simulink model "WiperSystem"  (R2023a)
settings: Solver=FixedStepDiscrete  StartTime=0.0  StopTime=20  FixedStep=0.001  RelTol=1e-3  EnableMultiTasking=on
undefined symbols (not defined in the file): sigbuilder_block
libraries: arduinolib x2, simulink x1
settings Model: ExtModeTrigDuration=2  Creator=waleed.elshemy  LastModifiedBy=Youssef Ait Mouna
settings SolverCC: AutoInsertRateTranBlk=on
settings OptimizationCC: UseDivisionForNetSlopeComputation=on  GainParamInheritBuiltInType=on  UseFloatMulNetSlope=on  PassReuseOutputArgsAs=Individual arguments  ZeroExternalMemoryAtStartup=off  ZeroInternalMemoryAtStartup=off  NoFixptDivByZeroProtection=on  EfficientFloat2IntCast=on  LifeSpan=1  MaxStackSize=64  OptimizeBlockOrder=speed  DifferentSizesBufferReuse=on  EfficientTunableParamExpr=on
settings DebuggingCC: ParameterTunabilityLossMsg=error  UnconnectedInputMsg=warning  UnconnectedOutputMsg=warning  UnconnectedLineMsg=warning
settings HardwareCC: ProdBitPerInt=16  ProdBitPerPointer=16  ProdBitPerSizeT=16  ProdBitPerPtrDiffT=16  ProdLargestAtomicFloat=None  ProdWordSize=8  ProdHWDeviceType=Atmel->AVR
settings ModelReferenceCC: EnableRefExpFcnMdlSchedulingChecks=on
settings SFSimCC: MATLABDynamicMemAlloc=off
settings RTWCC: Description=Embedded Coder  SystemTargetFile=ert.tlc  HardwareBoard=Arduino Uno  TemplateMakefile=ert_default_tmf  Toolchain=Arduino AVR  BuildConfiguration=Faster Runs  DLArmComputeVersion=19.05
settings CodeAppCC: ForceParamTrailComments=on  IgnoreCustomStorageClasses=off  OperatorAnnotations=on  SimulinkDataObjDesc=on  SFDataObjDesc=on  CustomSymbolStrGlobalVar=rt$N$M  CustomSymbolStrType=$N$M  CustomSymbolStrFcn=$N$M$F  CustomSymbolStrMacro=$N$M  InsertBlockDesc=on
settings ERTTargetCC: IncludeMdlTerminateFcn=off  CombineSignalStateStructs=on  SupportComplex=off  SupportContinuousTime=on  SupportNonInlinedSFcns=on  SupportVariableSizeSignals=on  ExtModeTransport=3  ExtModeStaticAlloc=on  ExtModeAutomaticAllocSize=off  ExtModeStaticAllocSize=250  ExtModeMexFile=ext_xcp  ExtModeIntrfLevel=Level2 - Open  ERTFilePackagingFormat=CompactWithDataFile

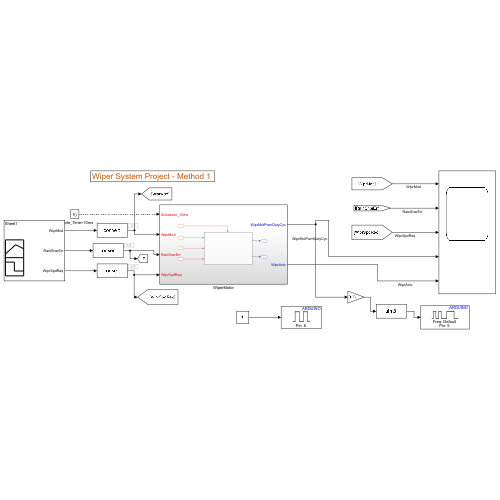
[thumbnail: Simulink's stored preview of the top-level diagram]
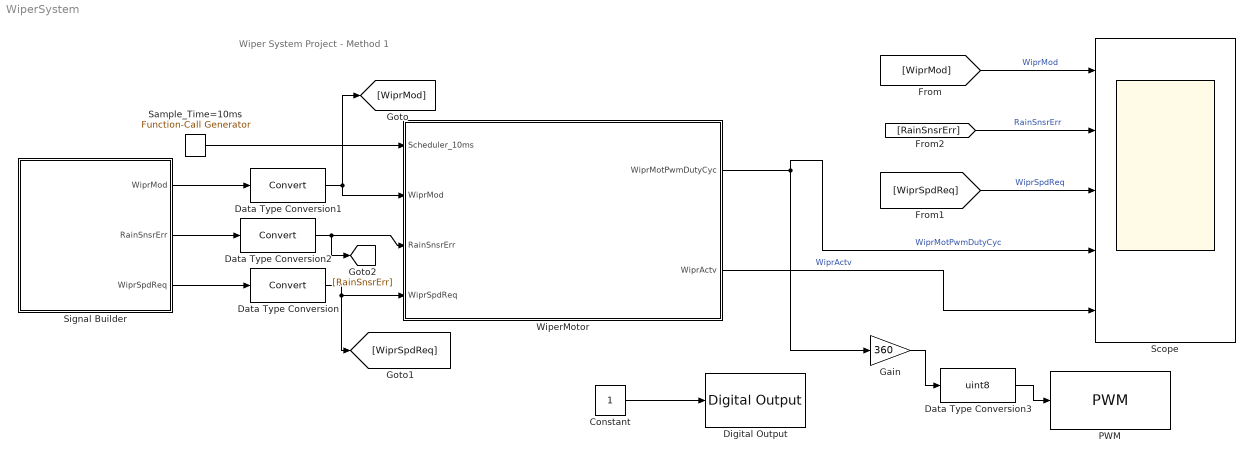
== system WiperSystem ==
  note: Wiper System Project - Method 1
  Constant : Constant
  Data Type Conversion : DataTypeConversion  SaturateOnIntegerOverflow=off  RndMeth=Floor
  Data Type Conversion1 : DataTypeConversion  SaturateOnIntegerOverflow=off  RndMeth=Floor
  Data Type Conversion2 : DataTypeConversion  SaturateOnIntegerOverflow=off  RndMeth=Floor
  Data Type Conversion3 : DataTypeConversion  OutDataTypeStr=uint8  SaturateOnIntegerOverflow=off  RndMeth=Floor
  Digital Output : arduinolib/Digital Output  pinNumber=6  Direction=output  blockPlatform=arduino
  Gain : Gain  Gain=360  OutDataTypeStr=uint8
  PWM : arduinolib/PWM  pinNumber=5  frequencyType=Default  desiredFrequency=490.2  achievableFrequency=490.2
  Sample_Time=10ms : simulink/Ports & Subsystems/Function-Call Generator  sample_time=0.01  numberOfIterations=1  DisallowWideOutput=off
  Scope : Scope  NumInputPorts=5
  Signal Builder : Subsystem  Tag=STV Subsys  LoadFcn=sigbuilder_block('load');  StartFcn=sigbuilder_block('start');  StopFcn=sigbuilder_block('stop');  ClipboardFcn=sigbuilder_block('clipboard');  mask(Sigbuilder block){tuvar=[0:10]}
      mask help: Simulink:masks:SigbuilderBlock_MD
      mask init:
      | if ~strcmp(get_param(bdroot(gcbh),'SimulationStatus'),'stopped') tuvar = sigbuilder_block('maskInit'); end
      settings: CopyFcn=sigbuilder_block('copy');  DeleteFcn=sigbuilder_block('delete');  ModelCloseFcn=sigbuilder_block('modelClose');  PreSaveFcn=sigbuilder_block('preSave');  PauseFcn=sigbuilder_block('pause');  ContinueFcn=sigbuilder_block('continue');  NameChangeFcn=sigbuilder_block('namechange');  OpenFcn=sigbuilder_block('open',[547.2 117.6 550.8 362.4 ]);  CloseFcn=sigbuilder_block('close');
      mask Display: plot(0, 0, 100, 100,[2, 2, 32, 32, 2], [68, 8, 8, 68, 68],[32, 2], [38, 38], [32, 19, 2],[53, 60, 44], [32, 17, 17, 2],[16, 16, 31, 31]);txt = getActiveGroup(gcbh);text(2, 100, txt,'verticalAlignment', 'top');
  WiperMotor : Subsystem
  wires:
  Sample_Time=10ms/1 -> WiperMotor/1(Scheduler_10ms)
  WiperMotor/1(WiprMotPwmDutyCyc) -> Scope/4, Gain/1  "WiprMotPwmDutyCyc"
  WiperMotor/2(WiprActv) -> Scope/5  "WiprActv"
  Signal Builder/1(WiprMod) -> Data Type Conversion1/1
  Signal Builder/3(WiprSpdReq) -> Data Type Conversion/1
  Data Type Conversion/1 -> [WiprSpdReq], WiperMotor/4(WiprSpdReq)
  Data Type Conversion1/1 -> [WiprMod], WiperMotor/2(WiprMod)
  [WiprMod] -> Scope/1  "WiprMod"
  Data Type Conversion2/1 -> [RainSnsrErr], WiperMotor/3(RainSnsrErr)
  Signal Builder/2(RainSnsrErr) -> Data Type Conversion2/1
  [WiprSpdReq] -> Scope/3  "WiprSpdReq"
  [RainSnsrErr] -> Scope/2  "RainSnsrErr"
  Constant/1 -> Digital Output/1
  Gain/1 -> Data Type Conversion3/1
  Data Type Conversion3/1 -> PWM/1

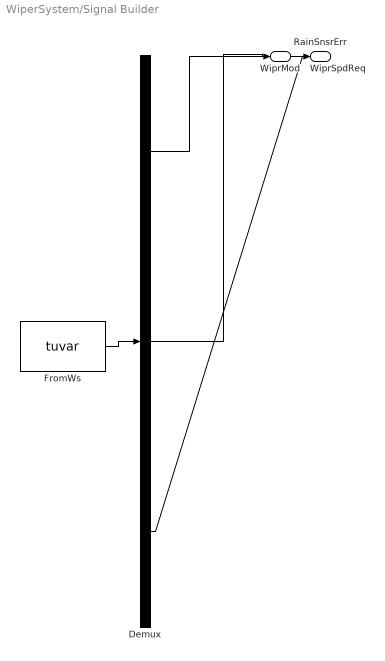
== system WiperSystem/Signal Builder ==
  Demux : Demux  Tag=STV Demux  Outputs=3
      settings: DisplayOption=none
  FromWs : FromWorkspace  Tag=STV FromWs  VariableName=tuvar  SampleTime=1  OutputAfterFinalValue=Holding final value
      SigBuilderData=|
      | common.afterFinalStr = 'Hold final value'
      | common.sampleTime = '1'
      | dataSet.timeRange = [0 16]
      | dataSet.name = 'Sheet1'
      | sbobj.Groups.Name = 'Sheet1'
      | sbobj.Groups.Signals(1).Name = 'WiprMod'
      | sbobj.Groups.Signals(1).XData = [0 1 2 3 4 5 6 7 8 9 10 11 12 13 14 15 16]
      | sbobj.Groups.Signals(1).YData = [0 0 2 2 3 3 1 1 1 1 1 1 1 1 1 1 1]
      | sbobj.Groups.Signals(2).Name = 'RainSnsrErr'
      | sbobj.Groups.Signals(2).XData = [0 1 2 3 4 5 6 7 8 9 10 11 12 13 14 15 16]
      | sbobj.Groups.Signals(2).YData = [0 0 0 0 0 0 0 0 0 0 0 0 0 0 0 1 0]
      | sbobj.Groups.Signals(3).Name = 'WiprSpdReq'
      | sbobj.Groups.Signals(3).XData = [0 1 2 3 4 5 6 7 8 9 10 11 12 13 14 15 16]
      | sbobj.Groups.Signals(3).YData = [0 0 0 0 0 0 0 0 1 2 3 4 5 6 7 7 7]
      | sbobj.Groups.TimeRange = [0 16]
  WiprMod : Outport  Tag=STV Outport
  RainSnsrErr : Outport  Tag=STV Outport  Port=2
  WiprSpdReq : Outport  Tag=STV Outport  Port=3
  wires:
  Demux/1 -> WiprMod/1
  FromWs/1 -> Demux/1
  Demux/2 -> RainSnsrErr/1
  Demux/3 -> WiprSpdReq/1

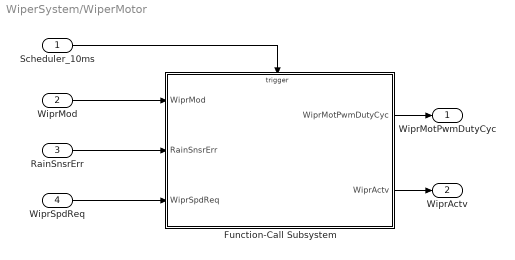
== system WiperSystem/WiperMotor ==
  Scheduler_10ms : Inport
  WiprMod : Inport  Port=2  OutMin=0  OutMax=3  OutDataTypeStr=uint8
  RainSnsrErr : Inport  Port=3  OutMin=0  OutMax=1  OutDataTypeStr=boolean
  WiprSpdReq : Inport  Port=4  OutMin=0  OutMax=7  OutDataTypeStr=uint8
  Function-Call Subsystem : Subsystem  TreatAsAtomicUnit=on
  WiprMotPwmDutyCyc : Outport  OutMin=0  OutMax=1  OutDataTypeStr=single  LockScale=on
  WiprActv : Outport  Port=2  OutDataTypeStr=boolean
  wires:
  WiprMod/1 -> Function-Call Subsystem/1(WiprMod)
  WiprSpdReq/1 -> Function-Call Subsystem/3(WiprSpdReq)
  Function-Call Subsystem/2(WiprActv) -> WiprActv/1
  Scheduler_10ms/1 -> Function-Call Subsystem/Trigger
  RainSnsrErr/1 -> Function-Call Subsystem/2(RainSnsrErr)
  Function-Call Subsystem/1(WiprMotPwmDutyCyc) -> WiprMotPwmDutyCyc/1

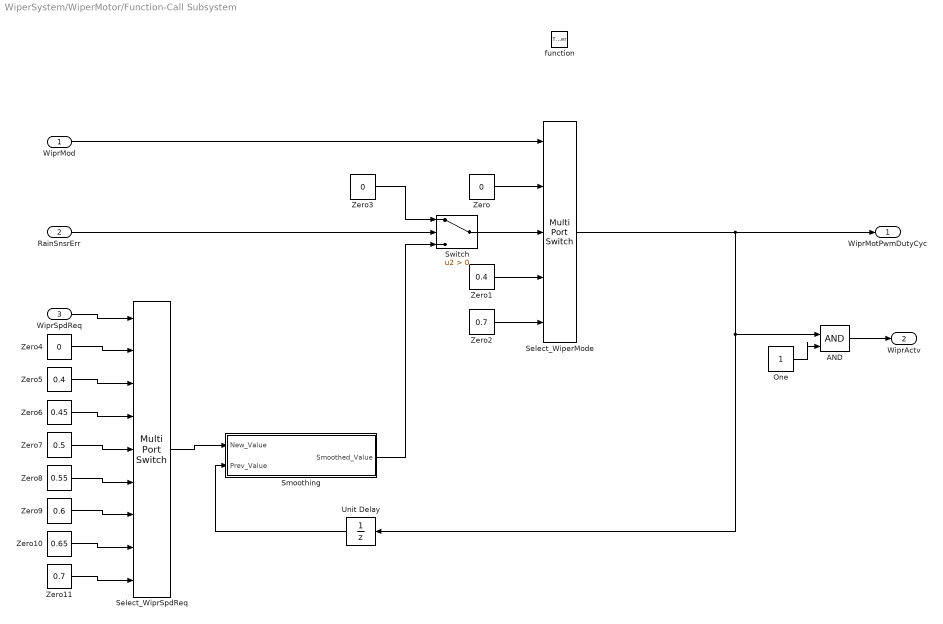
== system WiperSystem/WiperMotor/Function-Call Subsystem ==
  WiprMod : Inport
  RainSnsrErr : Inport  Port=2
  WiprSpdReq : Inport  Port=3
  function : TriggerPort  TriggerType=function-call  VariantControl=(inherit)
  AND : Logic  IconShape=distinctive  AllPortsSameDT=off  OutDataTypeStr=boolean
  One : Constant  OutDataTypeStr=Inherit: Inherit via back propagation
  Select_WiperMode : MultiPortSwitch  DataPortOrder=Zero-based contiguous  Inputs=4  zeroidx=on  OutDataTypeStr=single  SaturateOnIntegerOverflow=off  InputSameDT=off
  Select_WiprSpdReq : MultiPortSwitch  DataPortOrder=Zero-based contiguous  Inputs=8  zeroidx=on  SaturateOnIntegerOverflow=off  InputSameDT=off
  Smoothing : Subsystem
  Switch : Switch  Criteria=u2 > Threshold  OutDataTypeStr=single  SaturateOnIntegerOverflow=off  InputSameDT=off
  Unit Delay : UnitDelay  SampleTime=-1  HasFrameUpgradeWarning=on
  Zero : Constant  Value=0  OutDataTypeStr=Inherit: Inherit via back propagation
  Zero1 : Constant  Value=0.4  OutDataTypeStr=Inherit: Inherit via back propagation
  Zero10 : Constant  Value=0.65  OutDataTypeStr=Inherit: Inherit via back propagation
  Zero11 : Constant  Value=0.7  OutDataTypeStr=Inherit: Inherit via back propagation
  Zero2 : Constant  Value=0.7  OutDataTypeStr=Inherit: Inherit via back propagation
  Zero3 : Constant  Value=0  OutDataTypeStr=Inherit: Inherit via back propagation
  Zero4 : Constant  Value=0  OutDataTypeStr=Inherit: Inherit via back propagation
  Zero5 : Constant  Value=0.4  OutDataTypeStr=Inherit: Inherit via back propagation
  Zero6 : Constant  Value=0.45  OutDataTypeStr=Inherit: Inherit via back propagation
  Zero7 : Constant  Value=0.5  OutDataTypeStr=Inherit: Inherit via back propagation
  Zero8 : Constant  Value=0.55  OutDataTypeStr=Inherit: Inherit via back propagation
  Zero9 : Constant  Value=0.6  OutDataTypeStr=Inherit: Inherit via back propagation
  WiprMotPwmDutyCyc : Outport
  WiprActv : Outport  Port=2
  wires:
  WiprMod/1 -> Select_WiperMode/1
  Zero/1 -> Select_WiperMode/2
  Zero1/1 -> Select_WiperMode/4
  Zero2/1 -> Select_WiperMode/5
  Switch/1 -> Select_WiperMode/3
  RainSnsrErr/1 -> Switch/2
  Zero3/1 -> Switch/1
  Zero6/1 -> Select_WiprSpdReq/4
  Zero10/1 -> Select_WiprSpdReq/8
  Zero9/1 -> Select_WiprSpdReq/7
  WiprSpdReq/1 -> Select_WiprSpdReq/1
  Zero11/1 -> Select_WiprSpdReq/9
  Zero4/1 -> Select_WiprSpdReq/2
  Zero8/1 -> Select_WiprSpdReq/6
  Zero5/1 -> Select_WiprSpdReq/3
  Zero7/1 -> Select_WiprSpdReq/5
  Select_WiprSpdReq/1 -> Smoothing/1(New_Value)
  Select_WiperMode/1 -> Unit Delay/1, AND/1, WiprMotPwmDutyCyc/1
  AND/1 -> WiprActv/1
  Smoothing/1(Smoothed_Value) -> Switch/3
  Unit Delay/1 -> Smoothing/2(Prev_Value)
  One/1 -> AND/2

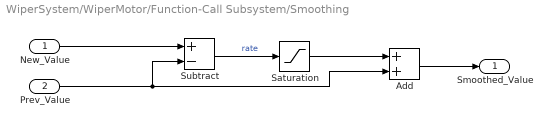
== system WiperSystem/WiperMotor/Function-Call Subsystem/Smoothing ==
  New_Value : Inport
  Prev_Value : Inport  Port=2
  Add : Sum
  Saturation : Saturate  UpperLimit=0.005  LowerLimit=-0.005
  Subtract : Sum  Inputs=+-
  Smoothed_Value : Outport
  wires:
  Prev_Value/1 -> Subtract/2, Add/2
  New_Value/1 -> Subtract/1
  Subtract/1 -> Saturation/1  "rate"
  Add/1 -> Smoothed_Value/1
  Saturation/1 -> Add/1
